simulink model "lowpassfilter_sim"  (R2023a)
settings: Solver=FixedStepAuto  StartTime=0.0  StopTime=10.0  FixedStep=Ts  RelTol=1e-3
values from neighbouring files (symbols this model uses):
  A = [a11, a12; a21, a22]    [dcmotor_ini.m]
  B = [b1; b2]    [dcmotor_ini.m]
  C = [w0*w0 0]    [dcmotor_ini.m]
  Ts = 1e-3    (= 0.001)    [dcmotor_ini.m]
settings Model: Creator=Michael Peter  LastModifiedBy=Michael Peter

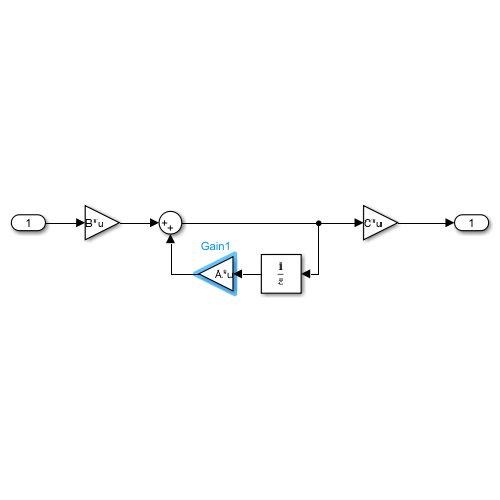
[thumbnail: Simulink's stored preview of the top-level diagram]
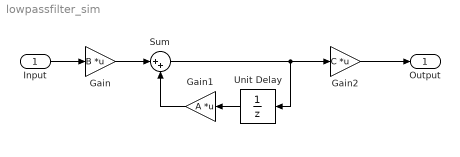
== system lowpassfilter_sim ==
  Input : Inport
  Gain : Gain  Gain=B  Multiplication=Matrix(K*u)
  Gain1 : Gain  Gain=A  Multiplication=Matrix(K*u)
  Gain2 : Gain  Gain=C  Multiplication=Matrix(K*u)
  Sum : Sum  Inputs=|++
  Unit Delay : UnitDelay  SampleTime=Ts  HasFrameUpgradeWarning=on
  Output : Outport
  wires:
  Gain/1 -> Sum/1
  Gain1/1 -> Sum/2
  Unit Delay/1 -> Gain1/1
  Sum/1 -> Gain2/1, Unit Delay/1
  Input/1 -> Gain/1
  Gain2/1 -> Output/1
